simulink model "scheme"  (R2016a)
settings: Solver=FixedStepAuto  StartTime=0.0  StopTime=inf  FixedStep=.01  MaxStep=.01  RelTol=1e-3
undefined symbols (not defined in the file or in its folder): transl
undefined symbols (not defined in the file): ctr
libraries: LibrarySimulinkSAS x5, simulink x3, dspfactors x1, simulink_extras x1, aerolibanimutils x1
settings Model: Creator=DSANTIAGO  LastModifiedBy=DSANTIAGO
settings DataIOCC: SaveOutput=off  SignalLogging=off  DSMLogging=off  SaveTime=off
settings OptimizationCC: DefaultUnderspecifiedDataType=single

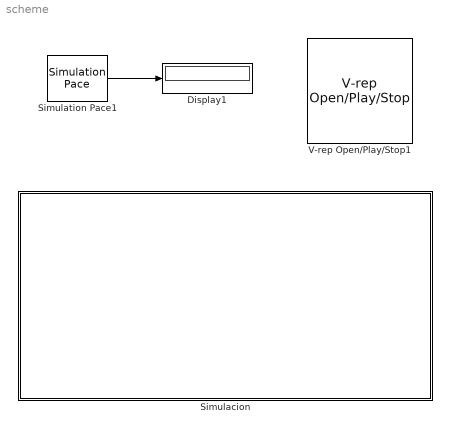
== system scheme ==
  Display1 : Display
  Simulacion : Subsystem  mask{sel=ctr, offSet=[1.8e-1 0 1.e-1]', h1=.01, h2=.01, kgmb=diag([8 10]), kgms=diag([5 5 5]), kms=15, kmb=5, ksb=1}
      mask prompts: sel "Control (s/m)"; h1 "Delay1"; h2 "Delay2"
  Simulation Pace1 : aerolibanimutils/Simulation Pace  SimulationPace=1  SleepMode=MATLAB Thread  OutputPaceError=on  SampleTime=-1
  V-rep Open/Play/Stop1 : LibrarySimulinkSAS/V-rep Open//Play//Stop  scene='escena_large.ttt'
  wires:
  Simulation Pace1/1 -> Display1/1

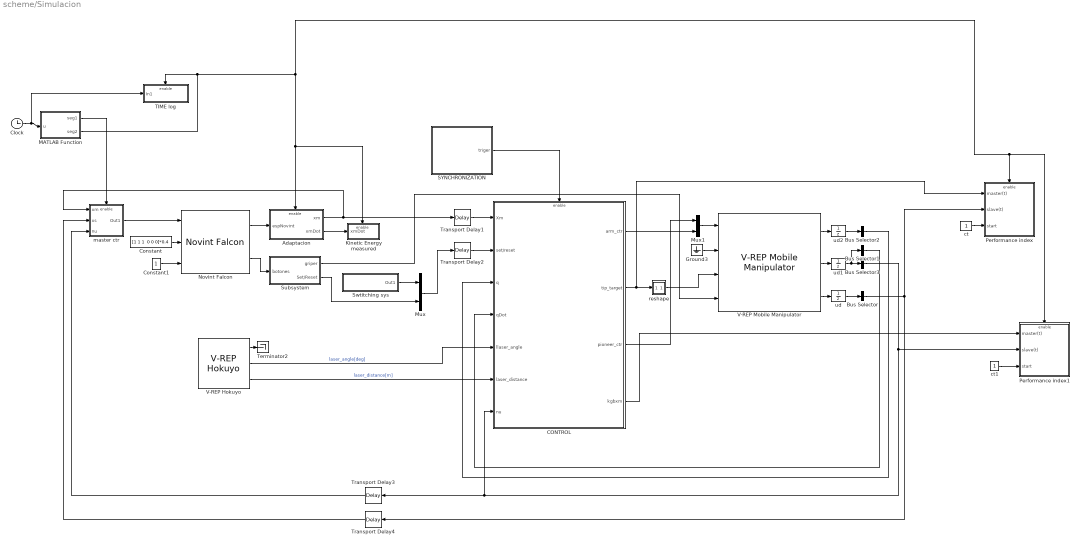
== system scheme/Simulacion ==
  Adaptacion : Subsystem
  Bus Selector : BusSelector  OutputSignals=xa,ya,za  OutputAsBus=on
  Bus Selector1 : BusSelector  OutputSignals=q1Dot,q2Dot,q3Dot,q4Dot  OutputAsBus=on
  Bus Selector2 : BusSelector  OutputSignals=q1,q2,q3,q4  OutputAsBus=on
  Bus Selector3 : BusSelector  OutputSignals=v,w  OutputAsBus=on
  CONTROL : Subsystem
  Clock : Clock
  Constant : Constant  Value="[1 1 1  0 0 0]*0.4"
  Constant1 : Constant  OutDataTypeStr=boolean
  Ground3 : Ground
  Kinetic Energy measured : Subsystem
  MATLAB Function : MATLAB Function  TreatAsAtomicUnit=on
  Mux : Mux  Inputs=2
  Mux1 : Mux  Inputs=2
  Novint Falcon : LibrarySimulinkSAS/Novint Falcon  dev=1
  Performance index : Subsystem
  Performance index1 : Subsystem
  SYNCHRONIZATION : Subsystem
  Subsystem : Subsystem
  Swtitching sys : Subsystem
  TIME log : Subsystem
  Terminator2 : Terminator
  Transport Delay1 : TransportDelay  DelayTime=h1
  Transport Delay2 : TransportDelay  DelayTime=h1
  Transport Delay3 : TransportDelay  DelayTime=h2
  Transport Delay4 : TransportDelay  DelayTime=h2
  V-REP Hokuyo : LibrarySimulinkSAS/V-REP Hokuyo  id=3
  V-REP Mobile Manipulator : LibrarySimulinkSAS/V-REP Mobile Manipulator  id1=1  id2=2
  ct : Constant
  ct1 : Constant
  master ctr : Subsystem
  reshape : Subsystem
  ud : UnitDelay  SampleTime=-1
  ud1 : UnitDelay  SampleTime=-1
  ud2 : UnitDelay  SampleTime=-1
  wires:
  Transport Delay2/1 -> CONTROL/2(set/reset)
  master ctr/1(Out1) -> Novint Falcon/1
  Transport Delay1/1 -> CONTROL/1(Xm)
  Novint Falcon/1 -> Adaptacion/1(espNovint)
  Constant/1 -> Novint Falcon/2
  Constant1/1 -> Novint Falcon/3
  Adaptacion/2(xmDot) -> Kinetic Energy measured/1(xmDot)
  V-REP Hokuyo/1 -> Terminator2/1
  Adaptacion/1(xm) -> master ctr/1(xm), Transport Delay1/1
  Bus Selector2/1 -> CONTROL/3(q)
  Bus Selector1/1 -> CONTROL/4(qDot)
  V-REP Hokuyo/2 -> CONTROL/5(llaser_angle)  "laser_angle[deg]"
  V-REP Hokuyo/3 -> CONTROL/6(laser_distance)  "laser_distance[m]"
  CONTROL/2(tip_target) -> reshape/1(i), Performance index/1(master(t))
  SYNCHRONIZATION/1(triger) -> CONTROL/Enable
  Subsystem/1(griper) -> V-REP Mobile Manipulator/4
  ct/1 -> Performance index/3(start)
  reshape/1(o) -> V-REP Mobile Manipulator/3
  ct1/1 -> Performance index1/3(start)
  CONTROL/4(kgbxm) -> Performance index1/1(master(t))
  Mux/1 -> Transport Delay2/1
  Swtitching sys/1(Out1) -> Mux/1
  Transport Delay3/1 -> master ctr/3(nu)
  Transport Delay4/1 -> master ctr/2("xs ")
  Bus Selector3/1 -> Performance index1/2(slave(t)), CONTROL/7(nu), Transport Delay3/1
  Bus Selector/1 -> Performance index/2(slave(t)), Transport Delay4/1
  Novint Falcon/2 -> Subsystem/1(botones)
  Subsystem/2(Set/Reset) -> Mux/2
  Clock/1 -> TIME log/1(In1), MATLAB Function/1(u)
  MATLAB Function/2(seg2) -> Kinetic Energy measured/Enable, Adaptacion/Enable, Performance index1/Enable, Performance index/Enable, TIME log/Enable
  MATLAB Function/1(seg1) -> master ctr/Enable
  Ground3/1 -> V-REP Mobile Manipulator/2
  Mux1/1 -> V-REP Mobile Manipulator/1
  CONTROL/1(arm_ctr) -> Mux1/2
  CONTROL/3(pioneer_ctr) -> Mux1/1
  V-REP Mobile Manipulator/2 -> ud1/1
  V-REP Mobile Manipulator/1 -> ud2/1
  V-REP Mobile Manipulator/3 -> ud/1
  ud/1 -> Bus Selector/1
  ud1/1 -> Bus Selector1/1, Bus Selector3/1
  ud2/1 -> Bus Selector2/1

== system scheme/Simulacion/Adaptacion ==
  espNovint : Inport
  Enable : EnablePort
  Clock : Clock
  MATLAB Function : MATLAB Function  TreatAsAtomicUnit=on
  MATLAB Function1 : MATLAB Function  TreatAsAtomicUnit=on
  MATLAB Function2 : MATLAB Function  TreatAsAtomicUnit=on
  xm : Outport
  xmDot : Outport  Port=2
  wires:
  espNovint/1 -> MATLAB Function/1(u)
  MATLAB Function/1(y) -> MATLAB Function2/1(u), MATLAB Function1/1(u)
  MATLAB Function1/1(y) -> xm/1
  MATLAB Function2/1(y) -> xmDot/1
  Clock/1 -> MATLAB Function/2(clk)

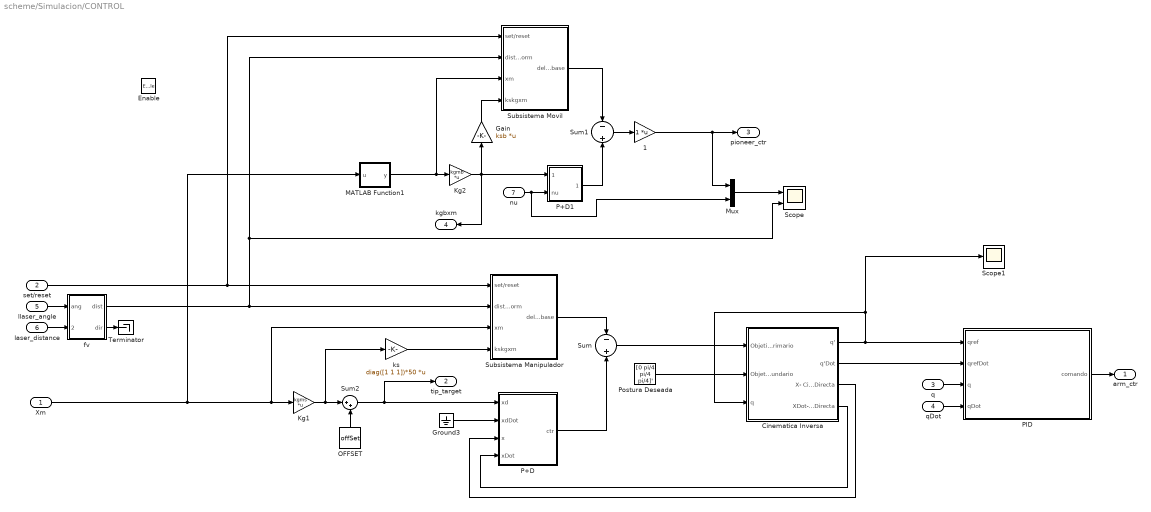
== system scheme/Simulacion/CONTROL ==
  Xm : Inport
  set/reset : Inport  Port=2
  q : Inport  Port=3
  qDot : Inport  Port=4
  llaser_angle : Inport  Port=5
  laser_distance : Inport  Port=6
  nu : Inport  Port=7
  Enable : EnablePort
  1 : Gain  Multiplication=Matrix(K*u)
  Cinematica Inversa : Subsystem
  Gain : Gain  Gain=ksb  Multiplication=Matrix(K*u)
  Ground3 : Ground
  Kg1 : Gain  Gain=kgms  Multiplication=Matrix(K*u)
  Kg2 : Gain  Gain=kgmb  Multiplication=Matrix(K*u)
  MATLAB Function1 : MATLAB Function  TreatAsAtomicUnit=on
  Mux : Mux  Inputs=2
  OFFSET : Constant  Value=offSet
  P+D : Subsystem
  P+D1 : Subsystem
  PID : Subsystem
  Postura Deseada : Constant  Value=[0 pi/4 pi/4 pi/4]'
  Scope : Scope  NumInputPorts=2
  Scope1 : Scope
  Subsistema Manipulador : Subsystem
  Subsistema Movil : Subsystem
  Sum : Sum  Inputs=-+
  Sum1 : Sum  Inputs=-+
  Sum2 : Sum  Inputs=|++
  Terminator : Terminator
  fv : Subsystem
  ks : Gain  Gain=diag([1 1 1])*50  Multiplication=Matrix(K*u)
  arm_ctr : Outport
  tip_target : Outport  Port=2
  pioneer_ctr : Outport  Port=3
  kgbxm : Outport  Port=4
  wires:
  Xm/1 -> Kg1/1, Subsistema Manipulador/3(xm), MATLAB Function1/1(u)
  Subsistema Manipulador/1(delta_base) -> Sum/1
  llaser_angle/1 -> fv/1(ang)
  laser_distance/1 -> fv/2(dist_in)
  Subsistema Movil/1(delta_base) -> Sum1/1
  P+D1/1(Out1) -> Sum1/2
  Kg2/1 -> kgbxm/1, Gain/1, P+D1/1(nu_ref)
  MATLAB Function1/1(y) -> Subsistema Movil/3(xm), Kg2/1
  q/1 -> PID/3(q)
  qDot/1 -> PID/4(qDot)
  Sum1/1 -> 1/1
  PID/1(comando) -> arm_ctr/1
  Cinematica Inversa/1(q') -> PID/1(qref), Scope1/1, Cinematica Inversa/3(q)
  Cinematica Inversa/2(q'Dot) -> PID/2(qrefDot)
  Postura Deseada/1 -> Cinematica Inversa/2(Objetivo Secundario)
  Ground3/1 -> P+D/2(xdDot)
  Cinematica Inversa/4(XDot- CinematicaDirecta) -> P+D/4(xDot)
  Sum2/1 -> P+D/1(xd), tip_target/1
  1/1 -> Mux/1, pioneer_ctr/1
  Cinematica Inversa/3(X- CinematicaDirecta) -> P+D/3(x)
  fv/1(dist) -> Subsistema Movil/2(dist_norm), Scope/2, Subsistema Manipulador/2(dist_norm)
  OFFSET/1 -> Sum2/2
  Kg1/1 -> ks/1, Sum2/1
  P+D/1(ctr) -> Sum/2
  Sum/1 -> Cinematica Inversa/1(Objetivo Primario)
  ks/1 -> Subsistema Manipulador/4(kskgxm)
  fv/2(dir) -> Terminator/1
  set/reset/1 -> Subsistema Movil/1(set/reset), Subsistema Manipulador/1(set/reset)
  nu/1 -> Mux/2, P+D1/2(nu)
  Gain/1 -> Subsistema Movil/4(kskgxm)
  Mux/1 -> Scope/1

== system scheme/Simulacion/Kinetic Energy measured ==
  xmDot : Inport
  Enable : EnablePort
  Display : Display
  Integrator : Integrator
  Kinetic Energy : MATLAB Function  TreatAsAtomicUnit=on
  To Workspace : ToWorkspace  VariableName=kinetic_energy  SampleTime=-1
  wires:
  Kinetic Energy/1(y) -> Integrator/1
  xmDot/1 -> Kinetic Energy/1(u)
  Integrator/1 -> Display/1, To Workspace/1

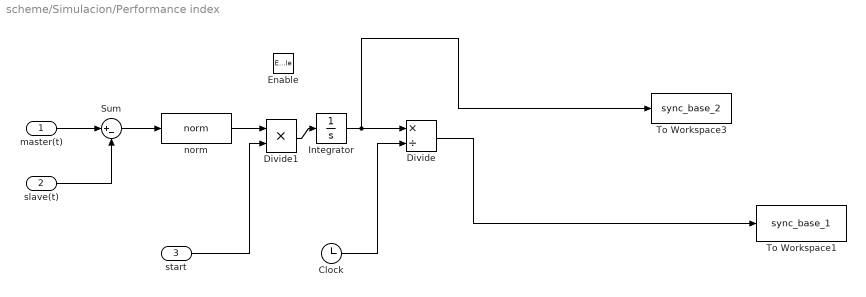
== system scheme/Simulacion/Performance index ==
  master(t) : Inport
  slave(t) : Inport  Port=2
  start : Inport  Port=3
  Enable : EnablePort
  Clock : Clock
  Divide : Product  Inputs=*/
  Divide1 : Product  Inputs=**
  Integrator : Integrator
  Sum : Sum  Inputs=|+-
  To Workspace1 : ToWorkspace  VariableName=sync_base_1  SampleTime=-1
  To Workspace3 : ToWorkspace  VariableName=sync_base_2  SampleTime=-1
  norm : MATLABFcn  MATLABFcn=norm
  wires:
  master(t)/1 -> Sum/1
  slave(t)/1 -> Sum/2
  Sum/1 -> norm/1
  Integrator/1 -> Divide/1, To Workspace3/1
  Divide/1 -> To Workspace1/1
  Clock/1 -> Divide/2
  norm/1 -> Divide1/1
  Divide1/1 -> Integrator/1
  start/1 -> Divide1/2

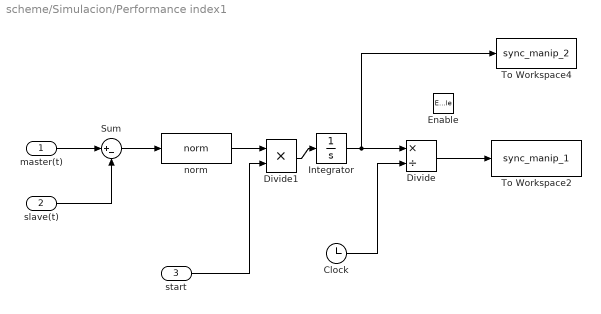
== system scheme/Simulacion/Performance index1 ==
  master(t) : Inport
  slave(t) : Inport  Port=2
  start : Inport  Port=3
  Enable : EnablePort
  Clock : Clock
  Divide : Product  Inputs=*/
  Divide1 : Product  Inputs=**
  Integrator : Integrator
  Sum : Sum  Inputs=|+-
  To Workspace2 : ToWorkspace  VariableName=sync_manip_1  SampleTime=-1
  To Workspace4 : ToWorkspace  VariableName=sync_manip_2  SampleTime=-1
  norm : MATLABFcn  MATLABFcn=norm
  wires:
  master(t)/1 -> Sum/1
  slave(t)/1 -> Sum/2
  Sum/1 -> norm/1
  Divide/1 -> To Workspace2/1
  Clock/1 -> Divide/2
  norm/1 -> Divide1/1
  Divide1/1 -> Integrator/1
  start/1 -> Divide1/2
  Integrator/1 -> Divide/1, To Workspace4/1

== system scheme/Simulacion/SYNCHRONIZATION ==
  MATLAB Function2 : MATLAB Function  TreatAsAtomicUnit=on
  Unit Delay : UnitDelay  SampleTime=-1
  Vrep-Count : LibrarySimulinkSAS/Simple Share Memory Block  nombre='vrep_counter'  dispositivo=5  vecE=[]  vecS=[1]  tipoE=[]  tipoS=['i']
  triger : Outport
  wires:
  Vrep-Count/1 -> MATLAB Function2/1(cnt_0), Unit Delay/1
  Unit Delay/1 -> MATLAB Function2/2(cnt_1)
  MATLAB Function2/1(y) -> triger/1

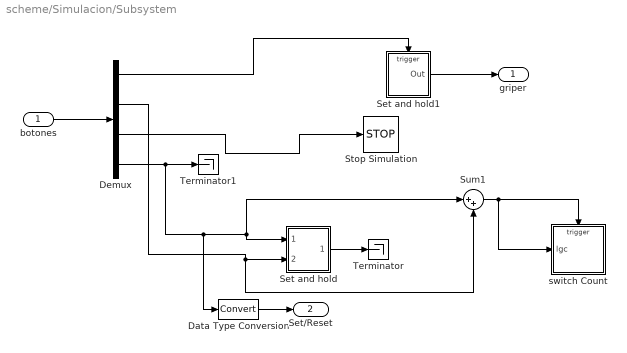
== system scheme/Simulacion/Subsystem ==
  botones : Inport
  Data Type Conversion : DataTypeConversion
  Demux : Demux
  Set and hold : Subsystem
  Set and hold1 : Subsystem
  Stop Simulation : Stop
  Sum1 : Sum  Inputs=|++
  Terminator : Terminator
  Terminator1 : Terminator
  switch Count : Subsystem
  griper : Outport
  Set/Reset : Outport  Port=2
  wires:
  botones/1 -> Demux/1
  Demux/3 -> Stop Simulation/1
  Demux/2 -> Sum1/2, Set and hold/2(reset)
  Demux/4 -> Data Type Conversion/1, Sum1/1, Set and hold/1(set), Terminator1/1
  Sum1/1 -> switch Count/1(lgc), switch Count/Trigger
  Data Type Conversion/1 -> Set/Reset/1
  Set and hold/1(Out) -> Terminator/1
  Set and hold1/1(Out) -> griper/1
  Demux/1 -> Set and hold1/Trigger

== system scheme/Simulacion/Swtitching sys ==
  Display : Display
  Keyboard 1 : M-S-Function  FunctionName=sfun_keyboard_input_v1_2b  mask(Keyboard Input){}
      mask help: Keyboard Input
      mask Display: fprintf('Keyboard');
  MATLAB Function : MATLAB Function  TreatAsAtomicUnit=on
  Mux : Mux  Inputs=2
  Terminator : Terminator
  Transfer Fcn1 : TransferFcn  Denominator=[.1 1]
  Transfer Fcn2 : TransferFcn  Denominator=[.1 1]
  Out1 : Outport
  wires:
  Keyboard 1/1 -> Display/1, MATLAB Function/1(u)
  MATLAB Function/2(m) -> Transfer Fcn1/1
  MATLAB Function/1(b) -> Transfer Fcn2/1
  Transfer Fcn1/1 -> Mux/2
  Transfer Fcn2/1 -> Mux/1
  Mux/1 -> Out1/1
  Keyboard 1/2 -> Terminator/1

== system scheme/Simulacion/TIME log ==
  In1 : Inport
  Enable : EnablePort
  To Workspace : ToWorkspace  VariableName=time  SampleTime=-1
  wires:
  In1/1 -> To Workspace/1

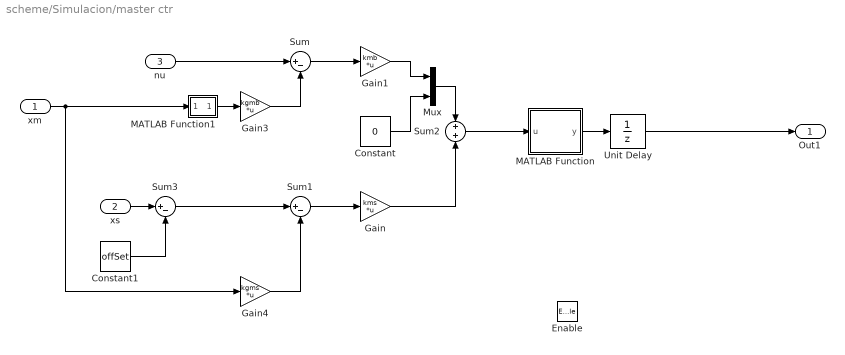
== system scheme/Simulacion/master ctr ==
  xm : Inport
  "xs " : Inport  Port=2
  nu : Inport  Port=3
  Enable : EnablePort
  Constant : Constant  Value=0
  Constant1 : Constant  Value=offSet
  Gain : Gain  Gain=kms  Multiplication=Matrix(K*u)
  Gain1 : Gain  Gain=kmb  Multiplication=Matrix(K*u)
  Gain3 : Gain  Gain=kgmb  Multiplication=Matrix(K*u)
  Gain4 : Gain  Gain=kgms  Multiplication=Matrix(K*u)
  MATLAB Function : MATLAB Function  TreatAsAtomicUnit=on
  MATLAB Function1 : MATLAB Function  TreatAsAtomicUnit=on
  Mux : Mux  Inputs=2
  Sum : Sum  Inputs=|+-
  Sum1 : Sum  Inputs=|+-
  Sum2 : Sum
  Sum3 : Sum  Inputs=|+-
  Unit Delay : UnitDelay  SampleTime=-1
  Out1 : Outport
  wires:
  nu/1 -> Sum/1
  xm/1 -> MATLAB Function1/1(u), Gain4/1
  Sum/1 -> Gain1/1
  Sum1/1 -> Gain/1
  Gain1/1 -> Mux/1
  Gain/1 -> Sum2/2
  Sum2/1 -> MATLAB Function/1(u)
  Gain3/1 -> Sum/2
  Gain4/1 -> Sum1/2
  "xs "/1 -> Sum3/1
  Sum3/1 -> Sum1/1
  Constant1/1 -> Sum3/2
  Mux/1 -> Sum2/1
  Constant/1 -> Mux/2
  MATLAB Function/1(y) -> Unit Delay/1
  MATLAB Function1/1(y) -> Gain3/1
  Unit Delay/1 -> Out1/1

== system scheme/Simulacion/reshape ==
  i : Inport
  Constant : Constant  Value=[0 0 0]
  Mux : Mux  Inputs=2
  o : Outport
  wires:
  Mux/1 -> o/1
  Constant/1 -> Mux/2
  i/1 -> Mux/1

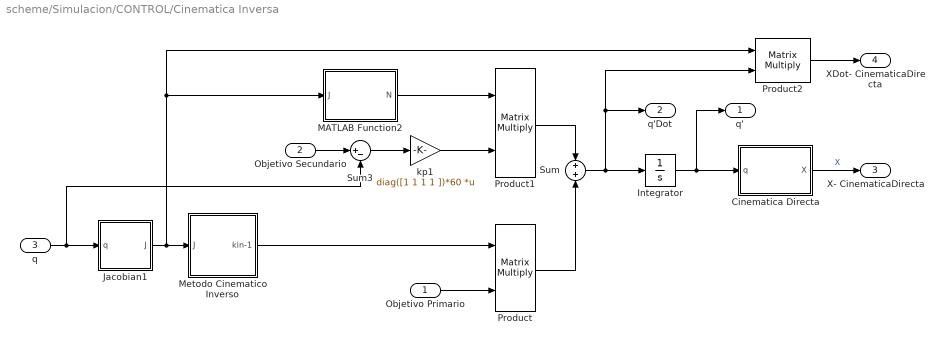
== system scheme/Simulacion/CONTROL/Cinematica Inversa ==
  Objetivo Primario : Inport
  Objetivo Secundario : Inport  Port=2
  q : Inport  Port=3
  Cinematica Directa : Subsystem
  Integrator : Integrator  InitialCondition=[.5 1 1 0]'*0  UpperSaturationLimit=[1 1 1 1]*2*pi  LowerSaturationLimit=-[1 1 1 1]*2*pi  WrapState=on
  Jacobian1 : Subsystem
  MATLAB Function2 : MATLAB Function  TreatAsAtomicUnit=on
  Metodo Cinematico Inverso : Subsystem
  Product : Product  Multiplication=Matrix(*)
  Product1 : Product  Multiplication=Matrix(*)
  Product2 : Product  Multiplication=Matrix(*)
  Sum : Sum
  Sum3 : Sum  Inputs=|+-
  kp1 : Gain  Gain=diag([1 1 1 1 ])*60  Multiplication=Matrix(K*u)
  q' : Outport
  q'Dot : Outport  Port=2
  X- CinematicaDirecta : Outport  Port=3
  XDot- CinematicaDirecta : Outport  Port=4
  wires:
  MATLAB Function2/1(N) -> Product1/1
  Product1/1 -> Sum/1
  Sum/1 -> Integrator/1, Product2/2, q'Dot/1
  Cinematica Directa/1("X ") -> X- CinematicaDirecta/1  "X"
  Product/1 -> Sum/2
  q/1 -> Sum3/2, Jacobian1/1(q)
  Jacobian1/1(J) -> MATLAB Function2/1(J), Product2/1, Metodo Cinematico Inverso/1(J)
  Objetivo Secundario/1 -> Sum3/1
  Sum3/1 -> kp1/1
  kp1/1 -> Product1/2
  Integrator/1 -> Cinematica Directa/1(q), q'/1
  Metodo Cinematico Inverso/1(kin-1) -> Product/1
  Objetivo Primario/1 -> Product/2
  Product2/1 -> XDot- CinematicaDirecta/1

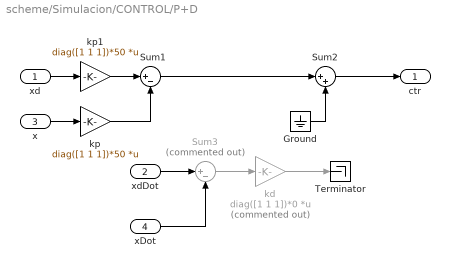
== system scheme/Simulacion/CONTROL/P+D ==
  xd : Inport
  xdDot : Inport  Port=2
  x : Inport  Port=3
  xDot : Inport  Port=4
  Ground : Ground
  Sum1 : Sum  Inputs=|+-
  Sum2 : Sum  Inputs=|++
  Sum3 : Sum  Commented=on  Inputs=|+-
  Terminator : Terminator
  kd : Gain  Commented=on  Gain=diag([1 1 1])*0  Multiplication=Matrix(K*u)
  kp : Gain  Gain=diag([1 1 1])*50  Multiplication=Matrix(K*u)
  kp1 : Gain  Gain=diag([1 1 1])*50  Multiplication=Matrix(K*u)
  ctr : Outport
  wires:
  x/1 -> kp/1
  xd/1 -> kp1/1
  Sum2/1 -> ctr/1
  xdDot/1 -> Sum3/1
  xDot/1 -> Sum3/2
  Sum3/1 -> kd/1
  kd/1 -> Terminator/1
  kp1/1 -> Sum1/1
  Sum1/1 -> Sum2/1
  kp/1 -> Sum1/2
  Ground/1 -> Sum2/2

== system scheme/Simulacion/CONTROL/P+D1 ==
  nu_ref : Inport
  nu : Inport  Port=2
  Manual Switch : ManualSwitch  Commented=on
  PID Controller : simulink/Continuous/PID Controller  Commented=on  Controller=PID  TimeDomain=Continuous-time  SampleTime=-1  IntegratorMethod=Forward Euler  FilterMethod=Forward Euler  Form=Parallel  UseFilter=on  ControllerParametersSource=internal  P=ksb  I=0  D=0  N=100  InitialConditionSource=internal  InitialConditionForIntegrator=0  InitialConditionForFilter=0  ExternalReset=none  LimitOutput=off  UpperSaturationLimit=inf  LowerSaturationLimit=-inf  LinearizeAsGain=on  AntiWindupMode=none  Kb=1  TrackingMode=off  Kt=1  PParamMin=[]  PParamMax=[]  IParamMin=[]  IParamMax=[]  DParamMin=[]  DParamMax=[]  NParamMin=[]  NParamMax=[]  KbParamMin=[]  KbParamMax=[]  KtParamMin=[]  KtParamMax=[]  POutMin=[]  POutMax=[]  IOutMin=[]  IOutMax=[]  DOutMin=[]  DOutMax=[]  NOutMin=[]  NOutMax=[]  KbOutMin=[]  KbOutMax=[]  KtOutMin=[]  KtOutMax=[]  IntegratorOutMin=[]  IntegratorOutMax=[]  FilterOutMin=[]  FilterOutMax=[]  SumOutMin=[]  SumOutMax=[]  SumI1OutMin=[]  SumI1OutMax=[]  SumI2OutMin=[]  SumI2OutMax=[]  SumI3OutMin=[]  SumI3OutMax=[]  SumDOutMin=[]  SumDOutMax=[]  SaturationOutMin=[]  SaturationOutMax=[]  IntegratorContinuousStateAttributes=''  IntegratorStateMustResolveToSignalObject=off  IntegratorRTWStateStorageClass=Auto  FilterContinuousStateAttributes=''  FilterStateMustResolveToSignalObject=off  FilterRTWStateStorageClass=Auto  DifferentiatorICPrevScaledInput=0  DifferentiatorOutMin=[]  DifferentiatorOutMax=[]
  Sum : Sum  Commented=on  Inputs=|+-
  Out1 : Outport
  wires:
  nu_ref/1 -> Out1/1
  nu/1 -> Sum/2
  Sum/1 -> PID Controller/1
  PID Controller/1 -> Manual Switch/2

== system scheme/Simulacion/CONTROL/PID ==
  note: En este esquema se esta utilizando el controlador Proporcional de Vrep
  qref : Inport
  qrefDot : Inport  Port=2
  q : Inport  Port=3
  qDot : Inport  Port=4
  Terminator : Terminator
  Terminator1 : Terminator
  Terminator2 : Terminator
  comando : Outport
  wires:
  qref/1 -> comando/1
  qrefDot/1 -> Terminator/1
  q/1 -> Terminator1/1
  qDot/1 -> Terminator2/1

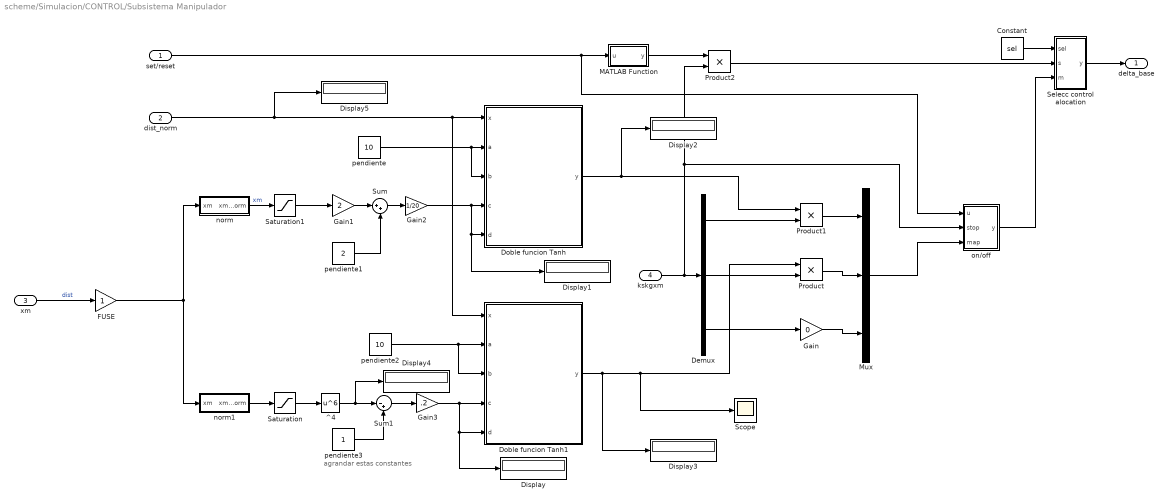
== system scheme/Simulacion/CONTROL/Subsistema Manipulador ==
  note: agrandar estas constantes
  set/reset : Inport
  dist_norm : Inport  Port=2
  xm : Inport  Port=3
  kskgxm : Inport  Port=4
  Constant : Constant  Value=sel
  Demux : Demux  Outputs=3
  Display{,1..5} (6 alike) : Display
  Doble funcion Tanh : MATLAB Function  TreatAsAtomicUnit=on
  Doble funcion Tanh1 : MATLAB Function  TreatAsAtomicUnit=on
  FUSE : Gain
  Gain : Gain  Gain=0
  Gain1 : Gain  Gain=2
  Gain2 : Gain  Gain=1/20
  Gain3 : Gain  Gain=.2
  MATLAB Function : MATLAB Function  TreatAsAtomicUnit=on
  Mux : Mux  Inputs=3
  Product : Product
  Product1 : Product
  Product2 : Product
  Saturation : Saturate  UpperLimit=1  LowerLimit=-1
  Saturation1 : Saturate  UpperLimit=1  LowerLimit=-1
  Scope : Scope
  Selecc control alocation : MATLAB Function  TreatAsAtomicUnit=on
  Sum : Sum  Inputs=|++
  Sum1 : Sum  Inputs=|-+
  ^4 : MATLABFcn  MATLABFcn=u^6
  norm : MATLAB Function  TreatAsAtomicUnit=on
  norm1 : MATLAB Function  TreatAsAtomicUnit=on
  on/off : MATLAB Function  TreatAsAtomicUnit=on
  pendiente : Constant  Value=10
  pendiente1 : Constant  Value=2
  pendiente2 : Constant  Value=10
  pendiente3 : Constant
  delta_base : Outport
  wires:
  kskgxm/1 -> on/off/2(stop), Product2/2, Demux/1
  Demux/3 -> Gain/1
  Demux/2 -> Product/2
  Demux/1 -> Product1/2
  Gain/1 -> Mux/3
  Product1/1 -> Mux/1
  Product/1 -> Mux/2
  dist_norm/1 -> Display5/1, Doble funcion Tanh1/1(x), Doble funcion Tanh/1(x)
  pendiente/1 -> Doble funcion Tanh/2(a), Doble funcion Tanh/3(b)
  norm/1(xm_norm) -> Saturation1/1  "xm"
  Sum/1 -> Gain2/1
  Gain1/1 -> Sum/1
  Gain2/1 -> Doble funcion Tanh/5(d), Display1/1, Doble funcion Tanh/4(c)
  Doble funcion Tanh/1(y) -> Display2/1, Product1/1
  pendiente1/1 -> Sum/2
  xm/1 -> FUSE/1  "dist"
  pendiente2/1 -> Doble funcion Tanh1/3(b), Doble funcion Tanh1/2(a)
  Gain3/1 -> Display/1, Doble funcion Tanh1/5(d), Doble funcion Tanh1/4(c)
  Doble funcion Tanh1/1(y) -> Display3/1, Scope/1, Product/1
  Sum1/1 -> Gain3/1
  pendiente3/1 -> Sum1/2
  ^4/1 -> Display4/1, Sum1/1
  norm1/1(xm_norm) -> Saturation/1
  Saturation/1 -> ^4/1
  Saturation1/1 -> Gain1/1
  Product2/1 -> Selecc control alocation/2(s)
  set/reset/1 -> on/off/1(u), MATLAB Function/1(u)
  MATLAB Function/1(y) -> Product2/1
  on/off/1(y) -> Selecc control alocation/3(m)
  Mux/1 -> on/off/3(map)
  Constant/1 -> Selecc control alocation/1(sel)
  Selecc control alocation/1(y) -> delta_base/1
  FUSE/1 -> norm/1(xm), norm1/1(xm)

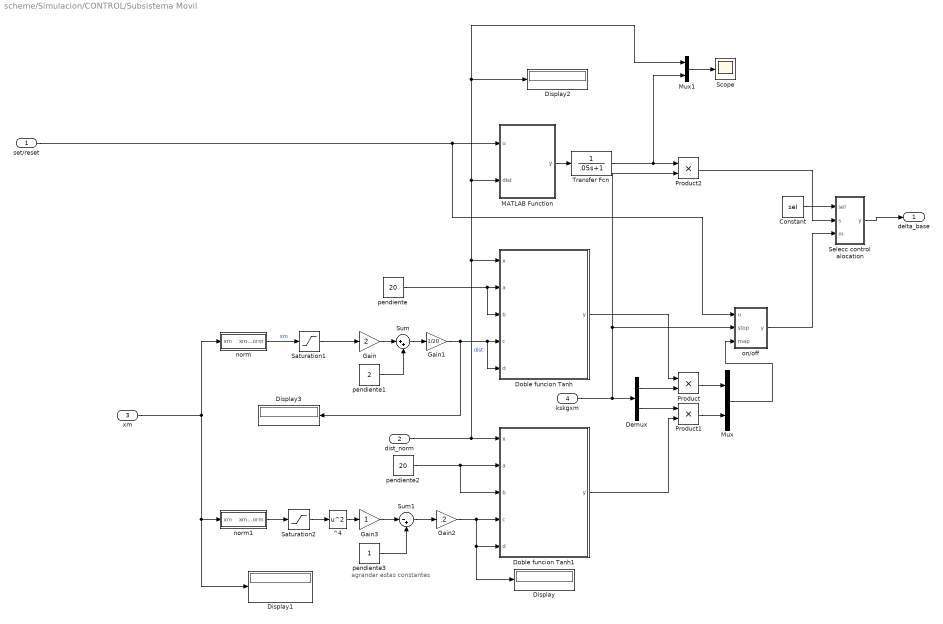
== system scheme/Simulacion/CONTROL/Subsistema Movil ==
  note: agrandar estas constantes
  set/reset : Inport
  dist_norm : Inport  Port=2
  xm : Inport  Port=3
  kskgxm : Inport  Port=4
  Constant : Constant  Value=sel
  Demux : Demux  Outputs=2
  Display{,1..3} (4 alike) : Display
  Doble funcion Tanh : MATLAB Function  TreatAsAtomicUnit=on
  Doble funcion Tanh1 : MATLAB Function  TreatAsAtomicUnit=on
  Gain : Gain  Gain=2
  Gain1 : Gain  Gain=1/20
  Gain2 : Gain  Gain=.2
  Gain3 : Gain
  MATLAB Function : MATLAB Function  TreatAsAtomicUnit=on
  Mux : Mux  Inputs=2
  Mux1 : Mux  Inputs=2
  Product : Product
  Product1 : Product
  Product2 : Product
  Saturation1 : Saturate  UpperLimit=1  LowerLimit=-1
  Saturation2 : Saturate  UpperLimit=1  LowerLimit=-1
  Scope : Scope
  Selecc control alocation : MATLAB Function  TreatAsAtomicUnit=on
  Sum : Sum  Inputs=|++
  Sum1 : Sum  Inputs=|-+
  Transfer Fcn : TransferFcn  Denominator=[.05 1]
  ^4 : MATLABFcn  MATLABFcn=u^2
  norm : MATLAB Function  TreatAsAtomicUnit=on
  norm1 : MATLAB Function  TreatAsAtomicUnit=on
  on/off : MATLAB Function  TreatAsAtomicUnit=on
  pendiente : Constant  Value=20
  pendiente1 : Constant  Value=2
  pendiente2 : Constant  Value=20
  pendiente3 : Constant
  delta_base : Outport
  wires:
  kskgxm/1 -> Demux/1, Product2/2, on/off/2(stop)
  Demux/1 -> Product/2
  Product/1 -> Mux/1
  Demux/2 -> Product1/1
  Product1/1 -> Mux/2
  Doble funcion Tanh/1(y) -> Product/1
  dist_norm/1 -> Doble funcion Tanh1/1(x), MATLAB Function/2(dist), Mux1/1, Display2/1, Doble funcion Tanh/1(x)  "dist"
  pendiente/1 -> Doble funcion Tanh/2(a), Doble funcion Tanh/3(b)
  norm/1(xm_norm) -> Saturation1/1  "xm"
  Sum/1 -> Gain1/1
  Gain/1 -> Sum/1
  pendiente1/1 -> Sum/2
  Gain1/1 -> Display3/1, Doble funcion Tanh/5(d), Doble funcion Tanh/4(c)
  pendiente2/1 -> Doble funcion Tanh1/2(a), Doble funcion Tanh1/3(b)
  Gain2/1 -> Display/1, Doble funcion Tanh1/5(d), Doble funcion Tanh1/4(c)
  Doble funcion Tanh1/1(y) -> Product1/2
  ^4/1 -> Gain3/1
  Sum1/1 -> Gain2/1
  pendiente3/1 -> Sum1/2
  Gain3/1 -> Sum1/1
  norm1/1(xm_norm) -> Saturation2/1
  Saturation1/1 -> Gain/1
  Saturation2/1 -> ^4/1
  xm/1 -> Display1/1, norm1/1(xm), norm/1(xm)
  Selecc control alocation/1(y) -> delta_base/1
  Product2/1 -> Selecc control alocation/2(s)
  set/reset/1 -> on/off/1(u), MATLAB Function/1(u)
  MATLAB Function/1(y) -> Transfer Fcn/1
  Mux1/1 -> Scope/1
  Mux/1 -> on/off/3(map)
  on/off/1(y) -> Selecc control alocation/3(m)
  Constant/1 -> Selecc control alocation/1(sel)
  Transfer Fcn/1 -> Product2/1, Mux1/2

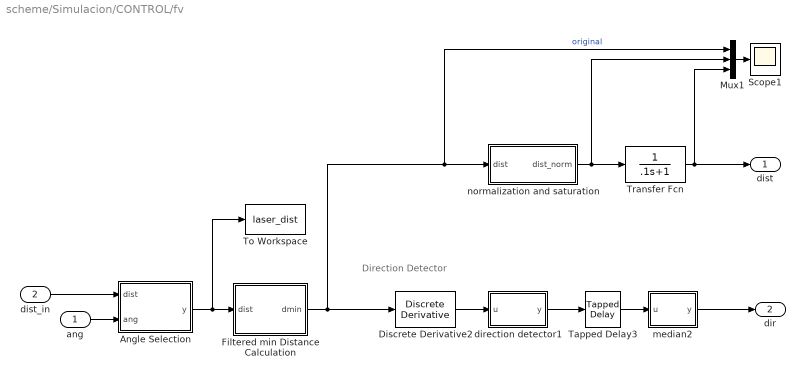
== system scheme/Simulacion/CONTROL/fv ==
  note: Direction Detector
  ang : Inport
  dist_in : Inport  Port=2
  Angle Selection : MATLAB Function  TreatAsAtomicUnit=on
  Discrete Derivative2 : simulink/Discrete/Discrete Derivative  gainval=1.0  ICPrevScaledInput=0.0  OutMin=[]  OutMax=[]  OutDataType=fixdt(1, 16)  OutScaling=2^-10  DoSatur=off
  Filtered min Distance Calculation : MATLAB Function  TreatAsAtomicUnit=on
  Mux1 : Mux  Inputs=3
  Scope1 : Scope
  Tapped Delay3 : simulink/Discrete/Tapped Delay  vinit=0.0  samptime=-1  NumDelays=6  DelayOrder=Oldest  includeCurrent=off
  To Workspace : ToWorkspace  VariableName=laser_dist  SampleTime=-1
  Transfer Fcn : TransferFcn  Denominator=[.1 1]
  direction detector1 : MATLAB Function  TreatAsAtomicUnit=on
  median2 : MATLAB Function  TreatAsAtomicUnit=on
  normalization and saturation : MATLAB Function  TreatAsAtomicUnit=on
  dist : Outport
  dir : Outport  Port=2
  wires:
  dist_in/1 -> Angle Selection/1(dist)
  Filtered min Distance Calculation/1(dmin) -> normalization and saturation/1(dist), Mux1/1, Discrete Derivative2/1  "original"
  Discrete Derivative2/1 -> direction detector1/1(u)
  direction detector1/1(y) -> Tapped Delay3/1
  median2/1(y) -> dir/1
  Tapped Delay3/1 -> median2/1(u)
  ang/1 -> Angle Selection/2(ang)
  Angle Selection/1(y) -> To Workspace/1, Filtered min Distance Calculation/1(dist)
  normalization and saturation/1(dist_norm) -> Transfer Fcn/1, Mux1/2
  Mux1/1 -> Scope1/1
  Transfer Fcn/1 -> Mux1/3, dist/1

== system scheme/Simulacion/Subsystem/Set and hold ==
  set : Inport
  reset : Inport  Port=2
  Data Type Conversion : DataTypeConversion
  S-R Flip-Flop : simulink_extras/Flip Flops/S-R Flip-Flop  initial_condition=0
  Terminator1 : Terminator
  Out : Outport
  wires:
  Data Type Conversion/1 -> Out/1
  S-R Flip-Flop/1 -> Data Type Conversion/1
  set/1 -> S-R Flip-Flop/1
  S-R Flip-Flop/2 -> Terminator1/1
  reset/1 -> S-R Flip-Flop/2

== system scheme/Simulacion/Subsystem/Set and hold1 ==
  Trigger : TriggerPort  VariantControl=Variant  PortDimensions=1
  Data Type Conversion : DataTypeConversion
  MATLAB Function : MATLAB Function  TreatAsAtomicUnit=on
  Unit Delay : UnitDelay  SampleTime=-1
  Out : Outport
  wires:
  Data Type Conversion/1 -> Out/1
  MATLAB Function/1(y) -> Unit Delay/1, Data Type Conversion/1
  Unit Delay/1 -> MATLAB Function/1(M)

== system scheme/Simulacion/Subsystem/switch Count ==
  lgc : Inport
  Trigger : TriggerPort  VariantControl=Variant  PortDimensions=1
  Display : Display
  Sum : Sum  Inputs=|++
  To Workspace : ToWorkspace  VariableName=switch_cnt  SampleTime=-1
  Unit Delay : UnitDelay  SampleTime=-1
  wires:
  lgc/1 -> Sum/1
  Sum/1 -> Display/1, Unit Delay/1, To Workspace/1
  Unit Delay/1 -> Sum/2

== system scheme/Simulacion/CONTROL/Cinematica Inversa/Cinematica Directa ==
  q : Inport
  Mux1 : Mux  Inputs=3
  T2xyz1 : Subsystem
      mask help: Convert transform to xyz scalars
      mask Help:
      | Convert homogeneous transformation to position scalars.
      | 
      | 
      | <b>Inputs::</b>
      | 
      | T (4x4) a translation represented as a homogeneous transformation
      | 
      | <b>Outputs::</b>
      | 
      | x (1x1) x-coordinate
      | y (1x1) y-coordinate
      | z (1x1) z-coordinate
      | 
      | <b>Notes::</b>
      | 
      | - A wrapper for the Toolbox function transl().
  fkine : MATLAB Function  TreatAsAtomicUnit=on
  "X " : Outport
  wires:
  fkine/1(out1) -> T2xyz1/1(T)
  Mux1/1 -> "X "/1
  T2xyz1/1(x) -> Mux1/1
  T2xyz1/2(y) -> Mux1/2
  T2xyz1/3(z) -> Mux1/3
  q/1 -> fkine/1(in1)

== system scheme/Simulacion/CONTROL/Cinematica Inversa/Jacobian1 ==
  q : Inport
  MATLAB Function3 : MATLAB Function  TreatAsAtomicUnit=on
  Reshape : Reshape  OutputDimensionality=Row vector (2-D)
  jacob0 : MATLAB Function  TreatAsAtomicUnit=on
  J : Outport
  wires:
  q/1 -> Reshape/1
  MATLAB Function3/1(J) -> J/1
  Reshape/1 -> jacob0/1(in1)
  jacob0/1(out1) -> MATLAB Function3/1(Jc)

== system scheme/Simulacion/CONTROL/Cinematica Inversa/Metodo Cinematico Inverso ==
  J : Inport
  Inversa sin singularidad : Subsystem
  kin-1 : Outport
  wires:
  J/1 -> Inversa sin singularidad/1(J)
  Inversa sin singularidad/1(invJ) -> kin-1/1

== system scheme/Simulacion/CONTROL/Cinematica Inversa/Cinematica Directa/T2xyz1 ==
  T : Inport
  Demux : Demux  Outputs=3
  MATLAB Fcn : MATLABFcn  MATLABFcn=transl(u)  OutputDimensions=3
  x : Outport
  y : Outport  Port=2
  z : Outport  Port=3
  wires:
  T/1 -> MATLAB Fcn/1
  MATLAB Fcn/1 -> Demux/1
  Demux/1 -> x/1
  Demux/2 -> y/1
  Demux/3 -> z/1

== system scheme/Simulacion/CONTROL/Cinematica Inversa/Metodo Cinematico Inverso/Inversa sin singularidad ==
  note: Descompone la matriz en SVD y calcula la intersa de S luego recompone la matriz.
      | Si algun termino de la diagonal de S se acerca a 0 lo que hace es no calcular la inversa de ese valor.
      | En su lugar coloca la inversa en 0 (anula el grado de libertad singular)
  J : Inport
  Inversa Segura : MATLAB Function  TreatAsAtomicUnit=on
  Product : Product  Inputs=3  Multiplication=Matrix(*)
  Singular Value Decomposition1 : dspfactors/Singular Value Decomposition  wantv=on  wanterr=off
  transpose : MATLABFcn  MATLABFcn='  Output1D=off
  invJ : Outport
  wires:
  J/1 -> Singular Value Decomposition1/1
  Singular Value Decomposition1/2 -> Inversa Segura/1(u)
  Inversa Segura/1(y) -> Product/2
  Singular Value Decomposition1/1 -> transpose/1
  Product/1 -> invJ/1
  Singular Value Decomposition1/3 -> Product/1
  transpose/1 -> Product/3

== matlab function scheme/Simulacion/Adaptacion/MATLAB Function1 ==
  data: u input; y output
function y = fcn(u)
%#codegen

y = u(1:3);

== matlab function scheme/Simulacion/CONTROL/Cinematica Inversa/Jacobian1/MATLAB Function3 ==
  data: Jc input; J output
function J = Jaco(Jc)
J = Jc(1:3,:);

== matlab function scheme/Simulacion/Adaptacion/MATLAB Function ==
  data: u input; y output; clk input
function y = fcn(u,clk)
y=zeros(6,1);
y(1)= -u(3);%-1;  %x
y(2)= -u(1);    %y
y(3)=  u(2);    %z
y(4)= -u(4);
y(5)= -u(5);
y(6)=  u(6);
if(clk>1)
    y=y/100;%[cm->m]
else
    y=y*0;
end

== matlab function scheme/Simulacion/CONTROL/Cinematica Inversa/Metodo Cinematico Inverso/Inversa sin singularidad/Inversa Segura ==
  data: u input; y output
function y = fcn(u)

n=length(u);
invu=zeros(n,1);
for i=1:n
    if(abs(u(i))>0.005)
        invu(i)=1/u(i);
    else
        invu(i)=0;
    end
end

y=diag(invu);

== matlab function scheme/Simulacion/Adaptacion/MATLAB Function2 ==
  data: u input; y output
function y = fcn(u)
%#codegen

y = u(4:6);

== matlab function scheme/Simulacion/CONTROL/Subsistema Manipulador/Doble funcion Tanh ==
  data: x input; y output; a input; b input; c input; d input
function y   = gap(x,a,b,c,d)%chichon!
%a: pendiente positiva (parte negativa)
%b: pendiente negativa (parte positiva)
%Punto de corte pendiente Positiva= c/a
%Punto de corte pendiente Negativa= b/d
% Redefino los puntos para que corte en c y b 
c=c*a;
d=d*b;
c1=1/2*tanh(a*x+c);
c2=-1/2*tanh(b*x-d);
y = 1-(c1+c2);

== matlab function scheme/Simulacion/CONTROL/fv/direction detector1 ==
  data: u input; y output
function y = fcn(u)
if(u>0)
    y=-1;
elseif(u<0)
    y=1;
else
    y=0;
end

== matlab function scheme/Simulacion/CONTROL/fv/Angle Selection ==
  data: dist input; y output; ang input
function y = fcn(dist,ang)
max=90;
n=length(dist);
y=dist;
for i=1:n
    if( (abs(ang(i))>max) || (y(i)==0) )
        y(i)=2;
    end
end

== matlab function scheme/Simulacion/CONTROL/MATLAB Function1 ==
  data: u input; y output
function y = fcn(u)
%#codegen

y = u(1:2);

== matlab function scheme/Simulacion/CONTROL/Subsistema Movil/Doble funcion Tanh ==
  data: x input; y output; a input; b input; c input; d input
function y   = bump(x,a,b,c,d)%chichon!
%a: pendiente positiva (parte negativa)
%b: pendiente negativa (parte positiva)
%Punto de corte pendiente Positiva= c/a
%Punto de corte pendiente Negativa= b/d
% Redefino los puntos para que corte en c y b 
c=c*a;
d=d*b;
c1=1/2*tanh(a*x+c);
c2=-1/2*tanh(b*x-d);
y = c1+c2;

== matlab function scheme/Simulacion/CONTROL/Subsistema Movil/Doble funcion Tanh1 ==
  data: x input; y output; a input; b input; c input; d input
function y   = bump(x,a,b,c,d)%chichon!
%a: pendiente positiva (parte negativa)
%b: pendiente negativa (parte positiva)
%Punto de corte pendiente Positiva= c/a
%Punto de corte pendiente Negativa= b/d
% Redefino los puntos para que corte en c y b 
c=c*a;
d=d*b;
c1=1/2*tanh(a*x+c);
c2=-1/2*tanh(b*x-d);
y = c1+c2;

== matlab function scheme/Simulacion/CONTROL/Subsistema Movil/norm1 ==
  data: xm input; xm_norm output
function xm_norm = fcn(xm)
xm_max=0.054;
xm_norm=xm(2)/xm_max;

== matlab function scheme/Simulacion/CONTROL/fv/Filtered min Distance Calculation ==
  data: dmin output; dist input
%Funcion que busca el objeto mas cercano.
%Para estimar la distancia al objeto se toma una vecindad del punto minimo
%si no existen puntos consistentes con el minimo encontrado se elimina 
%y se busco el proximo minimo. 

function dmin  = fcn(dist)
win=10;%ventana en la que se buscan rayos sucesivos.
min_on_win=18;
delta=.01;
tries=1;
max=2;
dmin=max;
%busco un minimo consistente en todo el arreglo del laser
% el minimo es consistente si por lo menos 3 rayos sucesivos son similares
%si lo encuentro promedio los rayos similares.
%si no lo encuentro borro el minimo y vuelvo a buscar
%si recorri todo el arreglo y no encontre nada utilizo el maximo
n=length(dist);
while(tries<n)
    [min_dist,i]=min(dist);
    if i<win+1
        i=win+1;
    end
    accum=min_dist;
    k=1;
    for j=1:win
        if (i-j)>0 && (abs(dist(i-j)-min_dist)<delta)
            accum=accum+dist(i-j);
            k=k+1;
        end
        if(i+j)<n && (abs(dist(i+j)-min_dist)<delta)
            accum=accum+dist(i-j);
            k=k+1;
        end
    end
    if(k>min_on_win)
        dmin=accum/k;
        break
    else
        dist(i)=max;%elimino el falso minimo
    end
    tries=tries+1;
end
end

== matlab function scheme/Simulacion/CONTROL/Subsistema Movil/norm ==
  data: xm input; xm_norm output
function xm_norm = fcn(xm)
xm_max=0.05;
xm_norm=xm(1)/xm_max;

== matlab function scheme/Simulacion/CONTROL/fv/median2 ==
  data: u input; y output
function y = fcn(u)
y=median(u);

== matlab function scheme/Simulacion/SYNCHRONIZATION/MATLAB Function2 ==
  data: cnt_0 input; y output; cnt_1 input
function y = fcn(cnt_0,cnt_1)
if(cnt_0~=cnt_1)
    y=1;
else
    y=0;
end

== matlab function scheme/Simulacion/CONTROL/fv/normalization and saturation ==
  data: dist input; dist_norm output
function dist_norm = factor(dist)
%normaliza la distancia entre 1 y 0
max_dist=2; %distancia maxima tenida en cuenta
min_dist=.12; %distancia maxima de acercamiento
dist_norm=1;
if(dist<max_dist)
    dist_norm=dist/max_dist;%normalizacion
end
% if(dist<min_dist)
%     dist_norm=0;
% end

== matlab function scheme/Simulacion/CONTROL/Subsistema Manipulador/norm ==
  data: xm input; xm_norm output
function xm_norm = fcn(xm)
xm_max=0.05;
xm_norm=xm(1)/xm_max;

== matlab function scheme/Simulacion/CONTROL/Subsistema Manipulador/Doble funcion Tanh1 ==
  data: x input; y output; a input; b input; c input; d input
function y   = gap(x,a,b,c,d)%chichon!
%a: pendiente positiva (parte negativa)
%b: pendiente negativa (parte positiva)
%Punto de corte pendiente Positiva= c/a
%Punto de corte pendiente Negativa= b/d
% Redefino los puntos para que corte en c y b 
c=c*a;
d=d*b;
c1=1/2*tanh(a*x+c);
c2=-1/2*tanh(b*x-d);
y = 1-(c1+c2);

== matlab function scheme/Simulacion/CONTROL/Subsistema Manipulador/norm1 ==
  data: xm input; xm_norm output
function xm_norm = fcn(xm)
xm_max=0.054;
xm_norm=xm(2)/xm_max;

== matlab function scheme/Simulacion/CONTROL/Cinematica Inversa/MATLAB Function2 ==
  data: J input; N output
function N = Null(J)
Jp=pinv(J);
I=eye(length(J));
N=(I-Jp*J)';

== matlab function scheme/Simulacion/CONTROL/Subsistema Manipulador/MATLAB Function ==
  data: u input; y output
function y = soft_not(u)
y=1-u(2);

== matlab function scheme/Simulacion/Kinetic Energy measured/Kinetic Energy ==
  data: u input; y output
function y = fcn(u)
M=eye(3);
y = u'*M*u;

== matlab function scheme/Simulacion/Swtitching sys/MATLAB Function ==
  data: u input; b output; m output
function [b,m] = fcn(u)
b=0;
m=0;
if(u==97)
    b=1;
elseif(u==115)
    m=1;
end

== matlab function scheme/Simulacion/CONTROL/Subsistema Movil/MATLAB Function ==
  data: u input; y output; dist input
function y = fcn(u, dist)
b=u(1); %switching base 1: activa, 0 :inactiva
ni=1-u(3); %switching inpedancia: 1:activa 0: inactiva (NORMALMENTE ACTIVO)

if (ni<.5)&&(b>0.5) %si la impedancia esta inactiva
    y=0; %la base se libera
elseif (dist<=0.15) && (b>.5) %si estoy frente al objeto
    y=1; %freno
elseif (dist<=0.4) && (b>.5) %si estoy frente al objeto
   y=.5; %freno
else
    y=1-b; %la base depende del switching
end

== matlab function scheme/Simulacion/master ctr/MATLAB Function ==
  data: u input; y output
function y = fcn(u)
y = [-u(2);u(3);-u(1)];

== matlab function scheme/Simulacion/master ctr/MATLAB Function1 ==
  data: u input; y output
function y = fcn(u)

y = u(1:2);

== matlab function scheme/Simulacion/CONTROL/Subsistema Movil/on//off ==
  data: u input; y output; stop input; map input
function y = fc(u,stop,map)
if(u(1)>.5)
    y=map;
else
    y=stop;
end

== matlab function scheme/Simulacion/CONTROL/Subsistema Manipulador/on//off ==
  data: u input; y output; stop input; map input
function y = fc(u,stop,map)
if(u(1)>.5)
    y=map;
else
    y=stop;
end

== matlab function scheme/Simulacion/CONTROL/Subsistema Movil/Selecc control alocation ==
  data: sel input; y output; s input; m input
function y = fcn(sel,s,m)
if(sel==1)
    y = s;
else
    y=m;
end

== matlab function scheme/Simulacion/CONTROL/Subsistema Manipulador/Selecc control alocation ==
  data: sel input; y output; s input; m input
function y = fcn(sel,s,m)
if(sel==1)
    y = s;
else
    y=m;
end

== matlab function scheme/Simulacion/CONTROL/Cinematica Inversa/Jacobian1/jacob0 ==
  data: in1 input; out1 output
function out1 = jacob0(in1)
%#codegen

%    This function was generated by the Symbolic Math Toolbox version 6.1.
%    31-May-2017 14:13:46

q1 = in1(:,1);
q2 = in1(:,2);
q3 = in1(:,3);
q4 = in1(:,4);
t2 = q1+q2+q3+q4;
t3 = q1-q2-q3-q4;
t4 = q3+q4;
t5 = cos(t2);
t6 = t5.*(1.0./2.0);
t7 = cos(t3);
t8 = t7.*(1.0./2.0);
t9 = t6+t8;
t10 = cos(q4);
t11 = t10.*(1.0./5.0);
t12 = sin(q4);
t13 = sin(t2);
t14 = t13.*(1.0./2.0);
t15 = sin(t3);
t30 = t15.*(1.0./2.0);
t16 = t14-t30;
t17 = q2+q3+q4;
t18 = sin(t17);
t19 = t18.*(1.0./1.0e1);
t20 = q2+q3;
t21 = sin(t20);
t22 = t21.*(1.0./5.0);
t23 = sin(q2);
t24 = t23.*(1.0./5.0);
t25 = t19+t22+t24;
t26 = sin(t4);
t27 = t26.*(1.0./5.0);
t28 = t12.*(1.0./5.0);
t29 = t27+t28;
t31 = cos(t4);
t32 = t31.*(1.0./5.0);
t33 = t11+t32+1.0./1.0e1;
t34 = t14+t30;
t35 = t11+1.0./1.0e1;
t36 = t6-t8;
t37 = cos(t17);
t38 = sin(q1);
t39 = cos(q1);
out1 = reshape([-t25.*t38,t25.*t39,0.0,-t9.*t18+t16.*t37,-t18.*t34-t36.*t37,t18.^2+t37.^2,t9.*t33+t16.*t29,-t29.*t36+t33.*t34,-t18.*t33+t29.*t37,-t38,t39,0.0,t12.*t16.*(1.0./5.0)+t9.*t35,t12.*t36.*(-1.0./5.0)+t34.*t35,t12.*t37.*(1.0./5.0)-t18.*t35,-t38,t39,0.0,t5.*(1.0./2.0e1)+t7.*(1.0./2.0e1),t13.*(1.0./2.0e1)+t15.*(1.0./2.0e1),-t19,-t38,t39,0.0],[6, 4]);

== matlab function scheme/Simulacion/CONTROL/Cinematica Inversa/Cinematica Directa/fkine ==
  data: in1 input; out1 output
function out1 = fkine(in1)
%#codegen

%    This function was generated by the Symbolic Math Toolbox version 6.1.
%    31-May-2017 14:13:40

q1 = in1(1,:);
q2 = in1(2,:);
q3 = in1(3,:);
q4 = in1(4,:);
t2 = q1+q2+q3+q4;
t3 = q1-q2-q3-q4;
t4 = cos(t2);
t5 = cos(t3);
t6 = sin(t2);
t7 = sin(t3);
t8 = t7.*(1.0./2.0);
t9 = cos(q1);
t10 = sin(q1);
t11 = q2+q3+q4;
t12 = sin(t11);
t13 = q2+q3;
t14 = sin(t13);
t15 = t14.*2.0;
t16 = sin(q2);
t17 = t16.*2.0;
t18 = t12+t15+t17;
t19 = cos(t11);
out1 = reshape([t6.*(-1.0./2.0)+t8,t4.*(1.0./2.0)-t5.*(1.0./2.0),-t19,0.0,t4.*(-1.0./2.0)-t5.*(1.0./2.0),t6.*(-1.0./2.0)-t8,t12,0.0,-t10,t9,0.0,0.0,t9.*t18.*(1.0./1.0e1),t10.*t18.*(1.0./1.0e1),t19.*(1.0./1.0e1)+cos(q2).*(1.0./5.0)+cos(t13).*(1.0./5.0)+1.0./5.0,1.0],[4, 4]);

== matlab function scheme/Simulacion/Subsystem/Set and hold1/MATLAB Function ==
  data: M input; y output
function y = fcn(M)
if(M==0)
    y=1;
else
    y=0;
end

== matlab function scheme/Simulacion/MATLAB Function ==
  data: u input; seg1 output; seg2 output
function [seg1,seg2] = fcn(u)
if(u>.5)
    seg1 = 1;
else
    seg1=0;
end
if(u>3)
    seg2 = 1;
else
    seg2=0;
end
